simulink library "ad_configsub"  (R2015b)
settings: Solver=ode45  StartTime=0.0  StopTime=10.0  RelTol=1e-3
values from neighbouring files (symbols this model uses):
  NTaps = 128    [Param_fir.m]
  Numerator = firls(NTaps-1, [0 Fpass Fstop Fs/2]/(Fs/2), [1 1 0 0], [Wpass Wstop])    [Param_fir.m]
libraries: hdlsllib x1, ad_configsub x1
settings Model: Creator=amatsumo  LastModifiedBy=amatsumo
settings DataIOCC: SaveFormat=Array  SignalLoggingSaveFormat=ModelDataLogs
settings OptimizationCC: ExpressionDepthLimit=2147483647
settings DebuggingCC: UnderspecifiedInitializationDetection=Classic  MergeDetectMultiDrivingBlocksExec=none  SolverPrmCheckMsg=warning  FcnCallInpInsideContextMsg=UseLocalSettings  StateNameClashWarn=warning  StrictBusMsg=Warning
settings HardwareCC: ProdBitPerPointer=32  ProdLargestAtomicFloat=None  ProdIntDivRoundTo=Undefined  ProdEndianess=Unspecified  ProdWordSize=32  ProdHWDeviceType=32-bit Generic
settings GRTTargetCC: GeneratePreprocessorConditionals=Disable all  CombineOutputUpdateFcns=off  GRTInterface=on
settings ConfigComp: CovModelRefEnable=Off  CovSFcnEnable=off

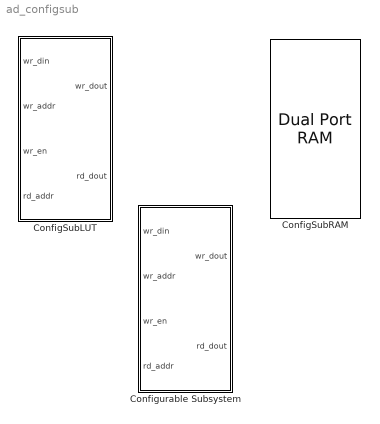
== system ad_configsub ==
  ConfigSubLUT : Subsystem
  ConfigSubRAM : hdlsllib/HDL Operations/Dual Port RAM  ram_size=ceil(log2(NTaps))
  Configurable Subsystem : Subsystem  BlockChoice=ConfigSubLUT
      settings: TemplateBlock=self  MemberBlocks=ConfigSubLUT,ConfigSubRAM

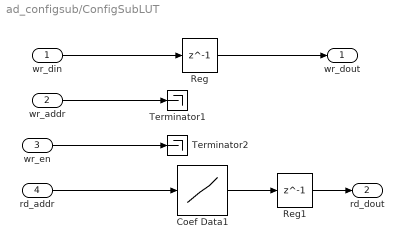
== system ad_configsub/ConfigSubLUT ==
  wr_din : Inport  OutDataTypeStr=fixdt('sfix16_En15')  PortDimensions=1  SampleTime=[7.8125000000000002e-005,0]
  wr_addr : Inport  Port=2  OutDataTypeStr=fixdt('ufix7')  PortDimensions=1  SampleTime=[7.8125000000000002e-005,0]
  wr_en : Inport  Port=3  OutDataTypeStr=boolean  PortDimensions=1  SampleTime=[7.8125000000000002e-005,0]
  rd_addr : Inport  Port=4  OutDataTypeStr=fixdt('ufix7')  PortDimensions=1  SampleTime=[7.8125000000000002e-005,0]
  Coef Data1 : Lookup  InputValues=[0:NTaps-1]  Table=Numerator  LookUpMeth=Use Input Nearest  OutDataTypeStr=fixdt(1,16,15)
  Reg : Delay  DelayLength=1  InputProcessing=Inherited
  Reg1 : Delay  DelayLength=1  InputProcessing=Inherited
  Terminator1 : Terminator
  Terminator2 : Terminator
  wr_dout : Outport  OutDataTypeStr=fixdt('sfix16_En15')  PortDimensions=1  SampleTime=[7.8125000000000002e-005,0]
  rd_dout : Outport  Port=2  OutDataTypeStr=fixdt('sfix16_En15')  PortDimensions=1  SampleTime=[7.8125000000000002e-005,0]
  wires:
  Reg1/1 -> rd_dout/1
  Reg/1 -> wr_dout/1
  wr_en/1 -> Terminator2/1
  rd_addr/1 -> Coef Data1/1
  wr_din/1 -> Reg/1
  wr_addr/1 -> Terminator1/1
  Coef Data1/1 -> Reg1/1

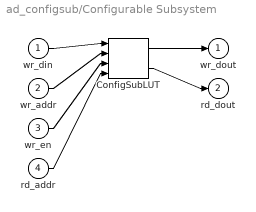
== system ad_configsub/Configurable Subsystem ==
  wr_din : Inport
  wr_addr : Inport  Port=2
  wr_en : Inport  Port=3
  rd_addr : Inport  Port=4
  ConfigSubLUT : ad_configsub/ConfigSubLUT
  wr_dout : Outport
  rd_dout : Outport  Port=2
  wires:
  wr_din/1 -> ConfigSubLUT/1
  wr_addr/1 -> ConfigSubLUT/2
  wr_en/1 -> ConfigSubLUT/3
  rd_addr/1 -> ConfigSubLUT/4
  ConfigSubLUT/1 -> wr_dout/1
  ConfigSubLUT/2 -> rd_dout/1
